simulink model "DegradationParameterRectifier"  (R2021a)
settings: Solver=VariableStepAuto  StartTime=0.0  StopTime=10.0  RelTol=1e-3
values from neighbouring files (symbols this model uses):
  rect_E1_M_adjustment = -0.1    [Run_GeneratorRectifierBoostConverterInverterMotorModel.m]    (also in Run_GeneratorRectifierBoostConverterModel.m; Run_GeneratorRectifierBuckConverterModel.m; Run_GeneratorRectifierModel.m)
  rect_f_sw_M_adjustment = -0.1    [Run_GeneratorRectifierBoostConverterInverterMotorModel.m]    (also in Run_GeneratorRectifierBoostConverterModel.m; Run_GeneratorRectifierBuckConverterModel.m; Run_GeneratorRectifierModel.m)
undefined symbols (not defined in the file or in its folder): rect_u_D_M_adjustment
libraries: Lib_EMTAT x4
settings Model: Creator=sfaulk  LastModifiedBy=mebell

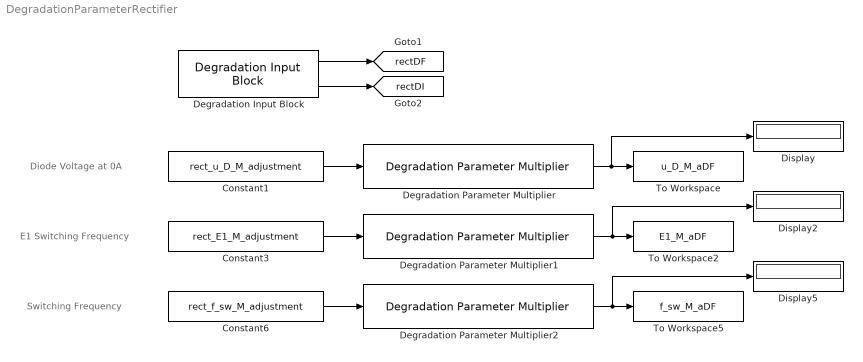
== system DegradationParameterRectifier ==
  note: Diode Voltage at 0A
  note: E1 Switching Frequency
  note: Switching Frequency
  Constant1 : Constant  Value=rect_u_D_M_adjustment
  Constant3 : Constant  Value=rect_E1_M_adjustment
  Constant6 : Constant  Value=rect_f_sw_M_adjustment
  Degradation Input Block : Lib_EMTAT/Components/Physics-Based/Degradation Input Block  SystemSampleTime=-1  VariantActivationTime=update diagram  Latency=0  AutoFrameSizeCalculation=off
      settings: SourceProductName=EMTAT
  Degradation Parameter Multiplier : Lib_EMTAT/Components/Physics-Based/Degradation Parameter Multiplier  SystemSampleTime=-1  VariantActivationTime=update diagram  Latency=0  AutoFrameSizeCalculation=off
      settings: SourceProductName=EMTAT
  Degradation Parameter Multiplier1 : Lib_EMTAT/Components/Physics-Based/Degradation Parameter Multiplier  SystemSampleTime=-1  VariantActivationTime=update diagram  Latency=0  AutoFrameSizeCalculation=off
      settings: SourceProductName=EMTAT
  Degradation Parameter Multiplier2 : Lib_EMTAT/Components/Physics-Based/Degradation Parameter Multiplier  SystemSampleTime=-1  VariantActivationTime=update diagram  Latency=0  AutoFrameSizeCalculation=off
      settings: SourceProductName=EMTAT
  Display : Display
  Display2 : Display
  Display5 : Display
  To Workspace : ToWorkspace  VariableName=u_D_M_aDF  SaveFormat=Timeseries  SampleTime=-1
      settings: Save2DSignal=2-D array (concatenate along first dimension)
  To Workspace2 : ToWorkspace  VariableName=E1_M_aDF  SaveFormat=Timeseries  SampleTime=-1
      settings: Save2DSignal=2-D array (concatenate along first dimension)
  To Workspace5 : ToWorkspace  VariableName=f_sw_M_aDF  SaveFormat=Timeseries  SampleTime=-1
      settings: Save2DSignal=2-D array (concatenate along first dimension)
  tag scope: rectDF=global, rectDI=global
  wires:
  Constant1/1 -> Degradation Parameter Multiplier/1
  Degradation Parameter Multiplier/1 -> Display/1, To Workspace/1
  Degradation Input Block/2 -> [rectDI]
  Degradation Input Block/1 -> [rectDF]
  Degradation Parameter Multiplier1/1 -> Display2/1, To Workspace2/1
  Constant3/1 -> Degradation Parameter Multiplier1/1
  Constant6/1 -> Degradation Parameter Multiplier2/1
  Degradation Parameter Multiplier2/1 -> Display5/1, To Workspace5/1
